simulink subsystem "Vehicle1D_measurement_refsub_logging"  (R2022a)
settings: Solver=VariableStepAuto  StartTime=0.0  StopTime=10.0  RelTol=1e-3
settings Model: Creator=isaacito  LastModifiedBy=isaacito

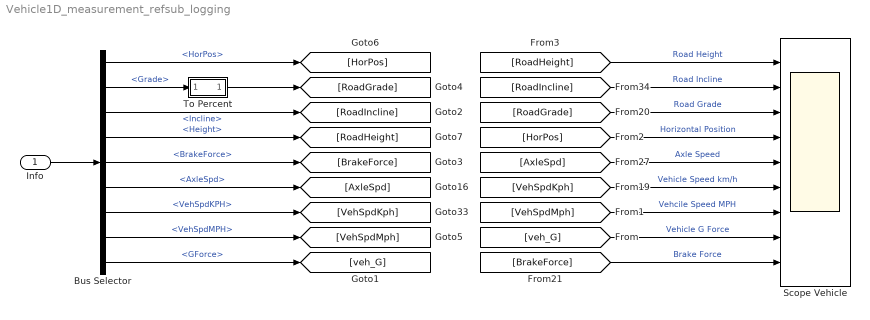
== system Vehicle1D_measurement_refsub_logging ==
  Info : Inport
  Bus Selector : BusSelector  OutputSignals=HorPos,Grade,Incline,Height,BrakeForce,AxleSpd,VehSpdKPH,VehSpdMPH,GForce
  Scope Vehicle : Scope  NumInputPorts=9
  To Percent : Subsystem
  wires:
  Bus Selector/9 -> [veh_G]  "<GForce>"
  Bus Selector/8 -> [VehSpdMph]  "<VehSpdMPH>"
  Bus Selector/7 -> [VehSpdKph]  "<VehSpdKPH>"
  Bus Selector/5 -> [BrakeForce]  "<BrakeForce>"
  Bus Selector/3 -> [RoadIncline]  "<Incline>"
  Info/1 -> Bus Selector/1
  Bus Selector/1 -> [HorPos]  "<HorPos>"
  Bus Selector/6 -> [AxleSpd]  "<AxleSpd>"
  Bus Selector/4 -> [RoadHeight]  "<Height>"
  [RoadHeight] -> Scope Vehicle/1  "Road Height"
  [RoadIncline] -> Scope Vehicle/2  "Road Incline"
  [RoadGrade] -> Scope Vehicle/3  "Road Grade"
  [HorPos] -> Scope Vehicle/4  "Horizontal Position"
  [AxleSpd] -> Scope Vehicle/5  "Axle Speed"
  [VehSpdKph] -> Scope Vehicle/6  "Vehicle Speed km/h"
  [VehSpdMph] -> Scope Vehicle/7  "Vehcile Speed MPH"
  [veh_G] -> Scope Vehicle/8  "Vehicle G Force"
  [BrakeForce] -> Scope Vehicle/9  "Brake Force"
  Bus Selector/2 -> To Percent/1(<Grade>)  "<Grade>"
  To Percent/1(Out1) -> [RoadGrade]

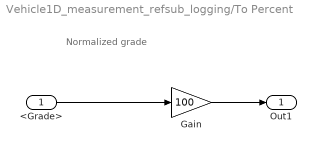
== system Vehicle1D_measurement_refsub_logging/To Percent ==
  note: Normalized grade
  <Grade> : Inport
  Gain : Gain  Gain=100
  Out1 : Outport  Unit=%
      settings: AttributesFormatString=%<Unit>
  wires:
  <Grade>/1 -> Gain/1
  Gain/1 -> Out1/1
